simulink model "kalman_oscillator_2021_03_27"  (R2020a)
settings: Solver=ode23tb  StartTime=0.0  StopTime=simlength  MaxStep=Ts
values from neighbouring files (symbols this model uses):
  Ad = [cos(w*Ts) sin(w*Ts); -sin(w*Ts) cos(w*Ts)]    [init_oscillator_2021_03_26.m]
  Afd = [exp(-Ts*w)*(1+Ts*w) exp(-Ts*w)*Ts; -exp(-Ts*w)*Ts*w^2 exp(-Ts*w)*(1-Ts*w)]    [init_oscillator_2021_03_26.m]
  Bfd = [(1-exp(-Ts*w)*(1+Ts*w))/w^2 exp(-Ts*w)*Ts]'    [init_oscillator_2021_03_26.m]
  C = [1 0]    [init_oscillator_2021_03_26.m]
  Cf = [2*w^2 0]    [init_oscillator_2021_03_26.m]
  pll_i1 = 2*pi/w    (= 0.004)    [init_oscillator_2021_03_26.m]
  pll_p = 2*pi/w    (= 0.004)    [init_oscillator_2021_03_26.m]
  Qkalman = [1 0; 0 1]*Ts    [init_oscillator_2021_03_26.m]
  Rkalman = 0.1/Ts    (= 2000)    [init_oscillator_2021_03_26.m]
  Tc = 1e-5    (= 1e-05)    [init_oscillator_2021_03_26.m]
  Ts = 1/20e3    (= 5e-05)    [init_oscillator_2021_03_26.m]
  w = 2*pi*f    (= 1570.79632679)    [init_oscillator_2021_03_26.m]
undefined symbols (not defined in the file or in its folder): magnitude
libraries: simulink x1
settings Model: SimulationMode=accelerator  Creator=dbagn  LastModifiedBy=dbagn
settings SolverCC: SolverResetMethod=Robust
settings DataIOCC: ReturnWorkspaceOutputs=off

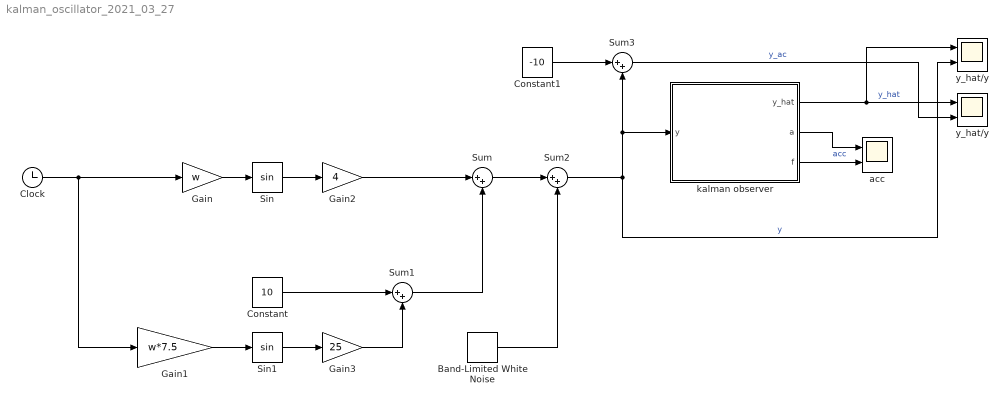
== system kalman_oscillator_2021_03_27 ==
  Band-Limited White Noise : simulink/Sources/Band-Limited White Noise  Cov=Tc  Ts=Tc  seed=[23341]
  Clock : Clock
  Constant : Constant  Value=10
  Constant1 : Constant  Value=-10
  Gain : Gain  Gain=w
  Gain1 : Gain  Gain=w*7.5
  Gain2 : Gain  Gain=4
  Gain3 : Gain  Gain=25
  Sin : Trigonometry
  Sin1 : Trigonometry
  Sum{,1..3} (4 alike) : Sum  Inputs=|++
  acc : Scope  NumInputPorts=2
  kalman observer : Subsystem
  y_hat/y : Scope  NumInputPorts=2
  "y_hat/y " : Scope  NumInputPorts=2
  wires:
  Gain/1 -> Sin/1
  kalman observer/1(y_hat) -> y_hat/y/1, "y_hat/y "/1  "y_hat"
  Sin/1 -> Gain2/1
  Sum1/1 -> Sum/2
  Gain1/1 -> Sin1/1
  Clock/1 -> Gain1/1, Gain/1
  Sin1/1 -> Gain3/1
  Gain2/1 -> Sum/1
  Sum/1 -> Sum2/1
  Sum2/1 -> "y_hat/y "/2, kalman observer/1(y), Sum3/2  "y"
  Constant/1 -> Sum1/1
  Band-Limited White Noise/1 -> Sum2/2
  kalman observer/2(a) -> acc/1  "acc"
  kalman observer/3(f) -> acc/2
  Gain3/1 -> Sum1/2
  Sum3/1 -> y_hat/y/2  "y_ac"
  Constant1/1 -> Sum3/1

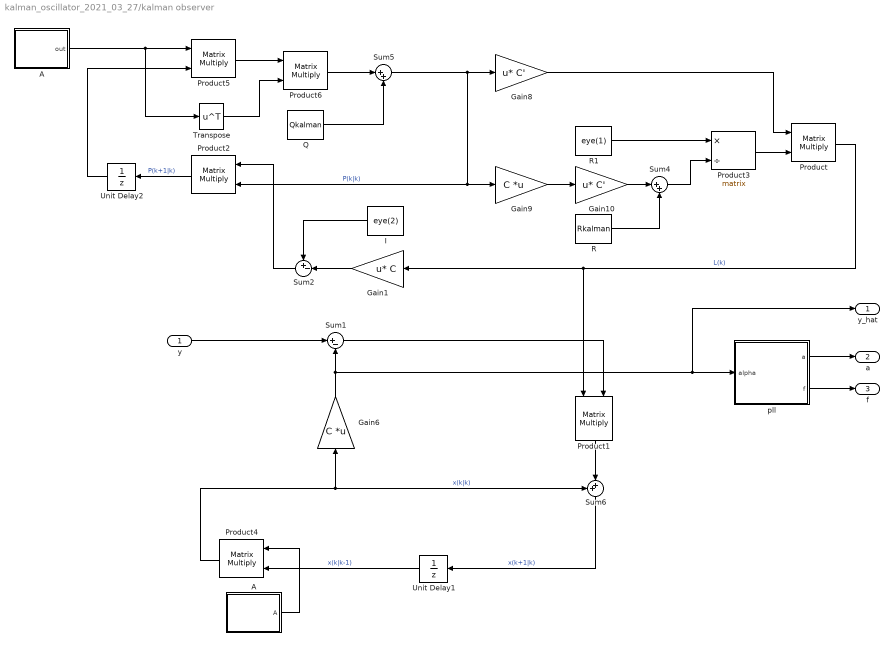
== system kalman_oscillator_2021_03_27/kalman observer ==
  y : Inport
  A : Subsystem
  "A " : Subsystem
  Gain1 : Gain  Gain=C  Multiplication=Matrix(u*K)
  Gain10 : Gain  Gain=C'  Multiplication=Matrix(u*K)
  Gain6 : Gain  Gain=C  Multiplication=Matrix(K*u)
  Gain8 : Gain  Gain=C'  Multiplication=Matrix(u*K)
  Gain9 : Gain  Gain=C  Multiplication=Matrix(K*u)
  I : Constant  Value=eye(2)
  Product{,1..2,4..6} (6 alike) : Product  Multiplication=Matrix(*)
  Product3 : Product  Inputs=*/  Multiplication=Matrix(*)
  Q : Constant  Value=Qkalman
  R : Constant  Value=Rkalman
  R1 : Constant  Value=eye(1)
  Sum1 : Sum  Inputs=|+-
  Sum2 : Sum  Inputs=+-|
  Sum4 : Sum  Inputs=|++
  Sum5 : Sum  Inputs=|++
  Sum6 : Sum  Inputs=++|
  Transpose : Math  Operator=transpose  SaturateOnIntegerOverflow=on
  Unit Delay1 : UnitDelay  InitialCondition=[0 0]  SampleTime=Ts  HasFrameUpgradeWarning=on
  Unit Delay2 : UnitDelay  SampleTime=Ts  HasFrameUpgradeWarning=on
  pll : Subsystem
  y_hat : Outport
  a : Outport  Port=2
  f : Outport  Port=3
  wires:
  Sum5/1 -> Product2/2, Gain9/1, Gain8/1  "P(k|k)"
  Product5/1 -> Product6/1
  Product6/1 -> Sum5/1
  Q/1 -> Sum5/2
  Gain9/1 -> Gain10/1
  R/1 -> Sum4/2
  Gain10/1 -> Sum4/1
  Gain8/1 -> Product/1
  Product/1 -> Product1/1, Gain1/1  "L(k)"
  Product2/1 -> Unit Delay2/1  "P(k+1|k)"
  Sum2/1 -> Product2/1
  Unit Delay2/1 -> Product5/2
  Sum6/1 -> Unit Delay1/1  "x(k+1|k)"
  I/1 -> Sum2/1
  Gain1/1 -> Sum2/2
  Sum1/1 -> Product1/2
  y/1 -> Sum1/1
  Sum4/1 -> Product3/2
  Product3/1 -> Product/2
  R1/1 -> Product3/1
  Product4/1 -> Gain6/1, Sum6/1  "x(k|k)"
  Unit Delay1/1 -> Product4/2  "x(k|k-1)"
  A/1(A) -> Product4/1
  "A "/1(out) -> Transpose/1, Product5/1
  Product1/1 -> Sum6/2
  Transpose/1 -> Product6/2
  Gain6/1 -> y_hat/1, pll/1(alpha), Sum1/2
  pll/1(a) -> a/1
  pll/2(f) -> f/1

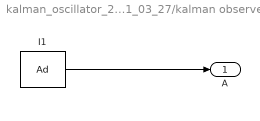
== system kalman_oscillator_2021_03_27/kalman observer/A ==
  I1 : Constant  Value=Ad
  A : Outport
  wires:
  I1/1 -> A/1

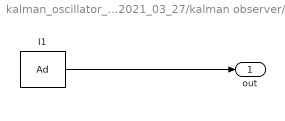
== system kalman_oscillator_2021_03_27/kalman observer/A  ==
  I1 : Constant  Value=Ad
  out : Outport
  wires:
  I1/1 -> out/1

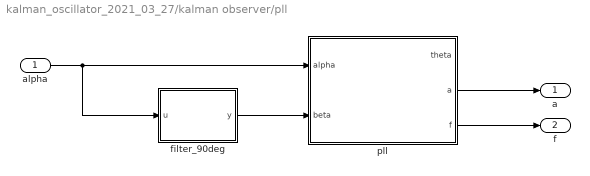
== system kalman_oscillator_2021_03_27/kalman observer/pll ==
  alpha : Inport
  filter_90deg : Subsystem
  pll : Subsystem
  a : Outport
  f : Outport  Port=2
  wires:
  pll/2(a) -> a/1
  pll/3(f) -> f/1
  alpha/1 -> filter_90deg/1(u), pll/1(alpha)
  filter_90deg/1(y) -> pll/2(beta)

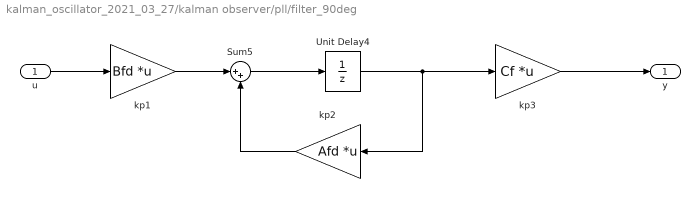
== system kalman_oscillator_2021_03_27/kalman observer/pll/filter_90deg ==
  u : Inport
  Sum5 : Sum  Inputs=|++
  Unit Delay4 : UnitDelay  SampleTime=Ts  HasFrameUpgradeWarning=on
  kp1 : Gain  Gain=Bfd  Multiplication=Matrix(K*u)  SaturateOnIntegerOverflow=on  OutDataTypeStr=Inherit: Same as input  ParamDataTypeStr=Inherit: Same as input
  kp2 : Gain  Gain=Afd  Multiplication=Matrix(K*u)  SaturateOnIntegerOverflow=on  OutDataTypeStr=Inherit: Same as input  ParamDataTypeStr=Inherit: Same as input
  kp3 : Gain  Gain=Cf  Multiplication=Matrix(K*u)  SaturateOnIntegerOverflow=on  OutDataTypeStr=Inherit: Same as input  ParamDataTypeStr=Inherit: Same as input
  y : Outport
  wires:
  Unit Delay4/1 -> kp2/1, kp3/1
  Sum5/1 -> Unit Delay4/1
  kp3/1 -> y/1
  kp2/1 -> Sum5/2
  kp1/1 -> Sum5/1
  u/1 -> kp1/1

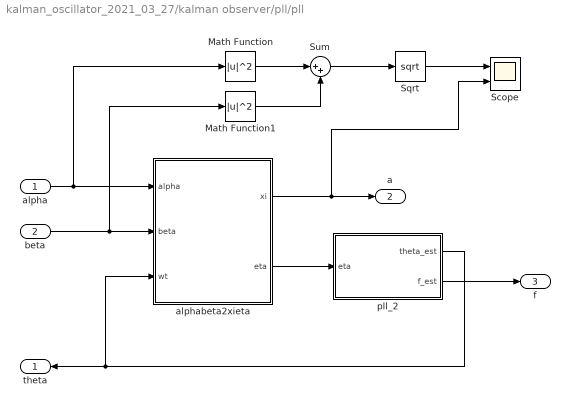
== system kalman_oscillator_2021_03_27/kalman observer/pll/pll ==
  alpha : Inport
  beta : Inport  Port=2
  Math Function : Math  Operator=magnitude^2  SaturateOnIntegerOverflow=on
  Math Function1 : Math  Operator=magnitude^2  SaturateOnIntegerOverflow=on
  Scope : Scope  NumInputPorts=2
  Sqrt : Sqrt  SaturateOnIntegerOverflow=on
  Sum : Sum  Inputs=|++
  alphabeta2xieta : Subsystem
  pll_2 : Subsystem
  theta : Outport
  a : Outport  Port=2
  f : Outport  Port=3
  wires:
  alpha/1 -> Math Function/1, alphabeta2xieta/1(alpha)
  beta/1 -> Math Function1/1, alphabeta2xieta/2(beta)
  pll_2/1(theta_est) -> alphabeta2xieta/3(wt), theta/1
  alphabeta2xieta/2(eta) -> pll_2/1(eta)
  alphabeta2xieta/1(xi) -> Scope/2, a/1
  pll_2/2(f_est) -> f/1
  Math Function/1 -> Sum/1
  Math Function1/1 -> Sum/2
  Sum/1 -> Sqrt/1
  Sqrt/1 -> Scope/1

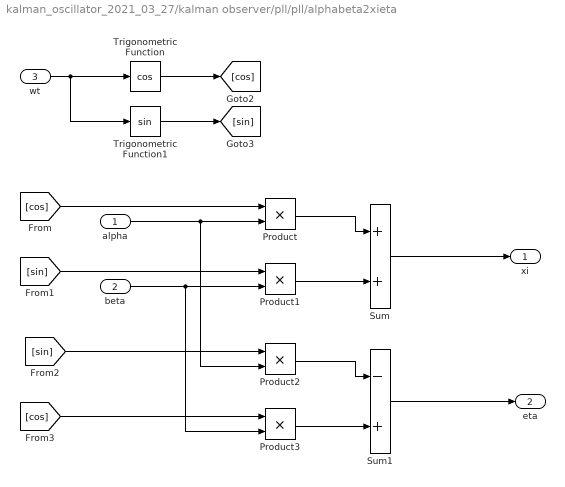
== system kalman_oscillator_2021_03_27/kalman observer/pll/pll/alphabeta2xieta ==
  alpha : Inport
  beta : Inport  Port=2
  wt : Inport  Port=3
  Product{,1..3} (4 alike) : Product  RndMeth=Zero
  Sum : Sum
  Sum1 : Sum  Inputs=-+
  Trigonometric Function : Trigonometry  Operator=cos
  Trigonometric Function1 : Trigonometry
  xi : Outport
  eta : Outport  Port=2
  wires:
  Trigonometric Function/1 -> [cos]
  Trigonometric Function1/1 -> [sin]
  wt/1 -> Trigonometric Function1/1, Trigonometric Function/1
  Sum1/1 -> eta/1
  Sum/1 -> xi/1
  [cos] -> Product3/1
  Product3/1 -> Sum1/2
  Product2/1 -> Sum1/1
  [sin] -> Product2/1
  beta/1 -> Product3/2, Product1/2
  [sin] -> Product1/1
  Product1/1 -> Sum/2
  Product/1 -> Sum/1
  alpha/1 -> Product2/2, Product/2
  [cos] -> Product/1

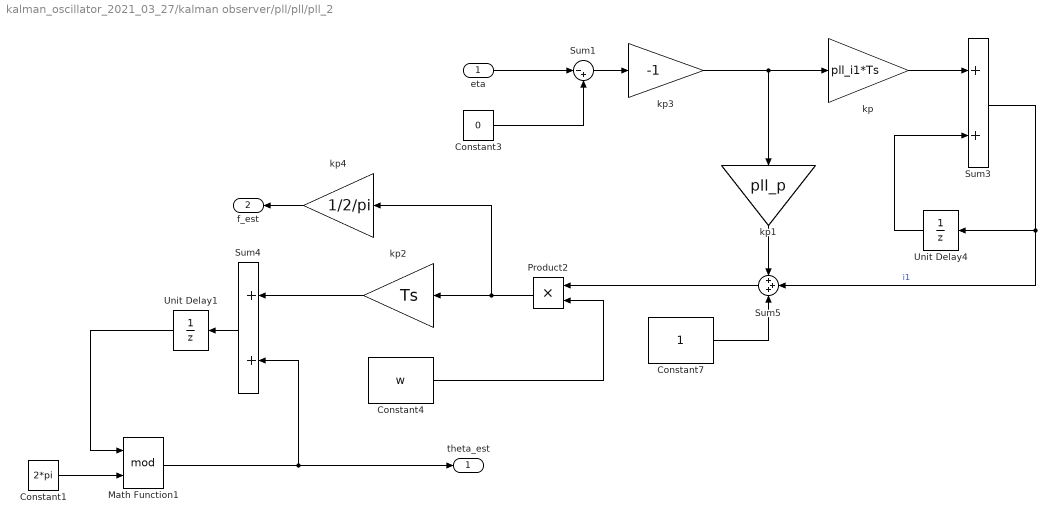
== system kalman_oscillator_2021_03_27/kalman observer/pll/pll/pll_2 ==
  eta : Inport
  Constant1 : Constant  Value=2*pi
  Constant3 : Constant  Value=0
  Constant4 : Constant  Value=w
  Constant7 : Constant
  Math Function1 : Math  Operator=mod  SignedPower=on  SaturateOnIntegerOverflow=on
  Product2 : Product  RndMeth=Zero
  Sum1 : Sum  Inputs=|-+
  Sum3 : Sum  SaturateOnIntegerOverflow=on
  Sum4 : Sum  SaturateOnIntegerOverflow=on
  Sum5 : Sum  Inputs=+++
  Unit Delay1 : UnitDelay  SampleTime=Ts  HasFrameUpgradeWarning=on
  Unit Delay4 : UnitDelay  SampleTime=Ts  HasFrameUpgradeWarning=on
  kp : Gain  Gain=pll_i1*Ts  SaturateOnIntegerOverflow=on  OutDataTypeStr=Inherit: Same as input  ParamDataTypeStr=Inherit: Same as input
  kp1 : Gain  Gain=pll_p  SaturateOnIntegerOverflow=on  OutDataTypeStr=Inherit: Same as input  ParamDataTypeStr=Inherit: Same as input
  kp2 : Gain  Gain=Ts  SaturateOnIntegerOverflow=on  OutDataTypeStr=Inherit: Same as input  ParamDataTypeStr=Inherit: Same as input
  kp3 : Gain  Gain=-1  SaturateOnIntegerOverflow=on  OutDataTypeStr=Inherit: Same as input  ParamDataTypeStr=Inherit: Same as input
  kp4 : Gain  Gain=1/2/pi  SaturateOnIntegerOverflow=on  OutDataTypeStr=Inherit: Same as input  ParamDataTypeStr=Inherit: Same as input
  theta_est : Outport
  f_est : Outport  Port=2
  wires:
  Constant3/1 -> Sum1/2
  Product2/1 -> kp4/1, kp2/1
  kp/1 -> Sum3/1
  Sum4/1 -> Unit Delay1/1
  kp1/1 -> Sum5/1
  eta/1 -> Sum1/1
  Sum1/1 -> kp3/1
  Sum3/1 -> Sum5/2, Unit Delay4/1  "i1"
  Unit Delay4/1 -> Sum3/2
  kp2/1 -> Sum4/1
  Sum5/1 -> Product2/1
  Constant4/1 -> Product2/2
  Math Function1/1 -> Sum4/2, theta_est/1
  Constant1/1 -> Math Function1/2
  kp3/1 -> kp/1, kp1/1
  kp4/1 -> f_est/1
  Constant7/1 -> Sum5/3
  Unit Delay1/1 -> Math Function1/1
